simulink model "ex2_2_3"  (R2023b)
settings: Solver=VariableStepAuto  StartTime=0.0  StopTime=10  RelTol=1e-3
libraries: simulink x2, dspsnks4 x1
settings Model: Creator=mariakahale  LastModifiedBy=mariakahale

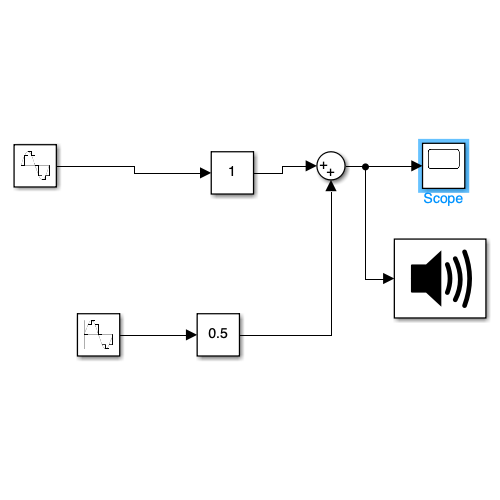
[thumbnail: Simulink's stored preview of the top-level diagram]
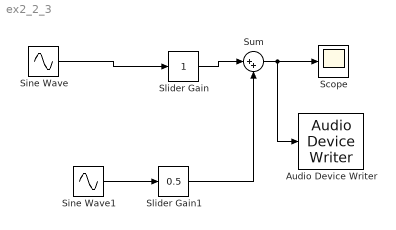
== system ex2_2_3 ==
  Audio Device Writer : dspsnks4/Audio Device Writer  Driver=CoreAudio  Device=Default  InheritSampleRate=on  SampleRate=44100  BitDepth=16-bit integer  BufferSize=4096  NumBuffers=10  DefaultOutputChannelMapping=on  OutputChannelMapping=1:2  OutputNumUnderrunSamples=off  DriverIdx=5  DeviceWarnFlag=''
  Scope : Scope
  Sine Wave : Sin  Frequency=6283  SampleTime=1/48000
  Sine Wave1 : Sin  Frequency=12566  SampleTime=1/48000
  Slider Gain : simulink/Math Operations/Slider Gain  gain=1  low=0  high=2
  Slider Gain1 : simulink/Math Operations/Slider Gain  gain=0.5  low=0  high=2
  Sum : Sum  Inputs=|++
  wires:
  Slider Gain/1 -> Sum/1
  Sum/1 -> Audio Device Writer/1, Scope/1
  Sine Wave/1 -> Slider Gain/1
  Sine Wave1/1 -> Slider Gain1/1
  Slider Gain1/1 -> Sum/2
